simulink model "sysgenPBDemo"  (Simulink 7.7)
settings: Solver=ode45  StartTime=0.0  StopTime=500  RelTol=1e-3
libraries: xbsIndex_r4 x19, xbsCopyrightNotice_r4 x1
settings Model: Creator=alexc  LastModifiedBy=arvinds
settings DataIOCC: SignalLoggingName=sigsOut
settings OptimizationCC: BooleanDataType=off  InlineInvariantSignals=on  InitFltsAndDblsToZero=on
settings DebuggingCC: SaveWithParameterizedLinksMsg=none  SignalResolutionControl=TryResolveAllWithWarning  SolverPrmCheckMsg=none  MultiTaskDSMMsg=warning  MultiTaskCondExecSysMsg=none  StrictBusMsg=None
settings HardwareCC: TargetUnknown=on
settings RTWCC: IncludeERTFirstTime=on
settings GRTTargetCC: TargetFcnLib=ansi_tfl_tmw.mat

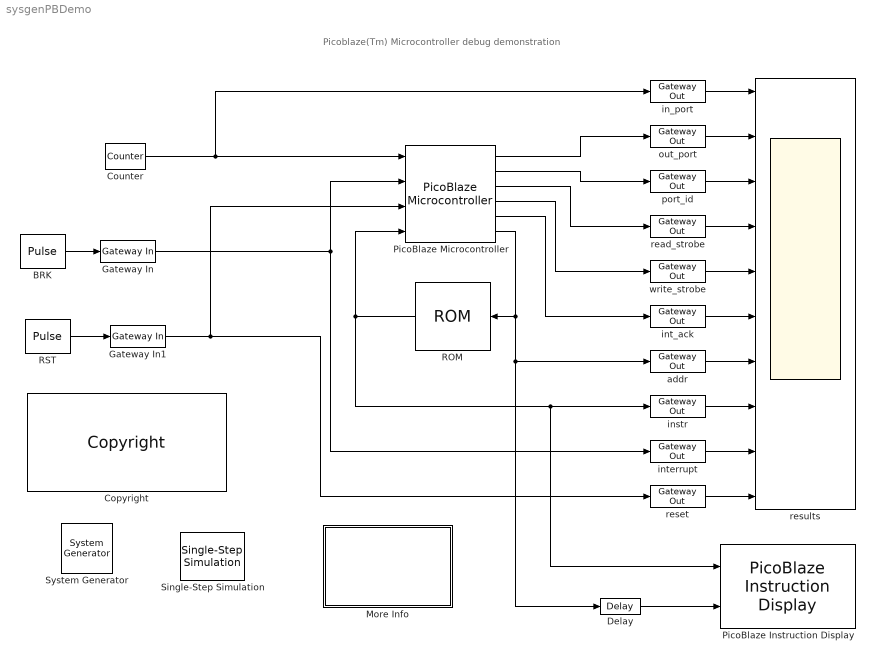
== system sysgenPBDemo ==
  note: Picoblaze(Tm) Microcontroller debug demonstration
  " System Generator" : xbsIndex_r4/ System Generator  Tag=genX  SystemSampleTime=-1  xilinxfamily=virtex4  part=xc4vlx200  speed=-11  package=ff1513  synthesis_tool=XST  clock_wrapper=Clock Enables  directory=C:/sb/demos/byhandtest/sysgenPBDemo  proj_type=Project Navigator  Synth_file=XST Defaults  Impl_file=ISE Defaults  testbench=on  simulink_period=1  sysclk_period=100  dcm_input_clock_period=100  incr_netlist=off  trim_vbits=Everywhere in SubSystem  dbl_ovrd=According to Block Masks  core_generation=According to Block Masks  run_coregen=off  deprecated_control=off  eval_field=0  block_type=sysgen
      settings: block_version=10.1.00
  BRK : DiscretePulseGenerator  Period=1000  PulseWidth=2
  Copyright : xbsCopyrightNotice_r4/Copyright  copyrighttext="Copyright (c) 2011  by  Xilinx, Inc. All rights reserved.<br><br>This file contains proprietary, confidential information of Xilinx, Inc., is distributed under license from Xilinx, Inc., and may be used, copied and/or disclosed only pursuant to the terms of a valid license agreement with Xilinx, Inc. Xilinx hereby grants you a license to use this file solely for design, simulation, implementation and creation of design files limited to Xilinx devices or technologies. Use with non-Xilinx devices or technologies is expressly prohibited and immediately terminates your license unless covered by a separate agreement.<br><br>Xilinx is providing this design, code, or information \"as-is\" solely for use in developing programs and solutions for Xilinx devices, with no obligation on the part of Xilinx to provide support. By providing this design, code, or information as one possible implementation of this feature, application or standard, Xilinx is making no representation that this implementation is free from any claims of infringement. You are responsible for obtaining any rights you may require for your implementation. Xilinx expressly disclaims any warranty whatsoever with respect to the adequacy of the implementation, including but not limited to any warranties or representations that this implementation is free from claims of infringement, implied warranties of merchantability or fitness for a particular purpose.<br><br>Xilinx products are not intended for use in life support appliances, devices, or systems. Use in such applications is expressly prohibited.<br><br>Any modifications that are made to the Source Code are done at the user's sole risk and will be unsupported.<br><br>This copyright and support notice must be retained as part of this text at all times. (c) Copyright 1995-2011 Xilinx, Inc. All rights reserved."  block_type=copyright
      settings: block_version=10.1.00
      settings: infoedit=|
      | Copyright(C) 2008 by  Xilinx, Inc. All rights reserved.<br>
      | <br>
      | This file contains proprietary, confidential information of Xilinx, Inc., is distributed under license
      | from Xilinx, Inc., and may be used, copied and/or disclosed only pursuant to the terms of a valid license
      | agreement with Xilinx, Inc. Xilinx hereby grants you a license to use this file solely for design,
      | simulation, implementation and creation of design files limited to Xilinx devices or technologies. Use
      | with non-Xilinx devices or technologies is expressly prohibited and immediately terminates your license
      | unless covered by a separate agreement.<br>
      | <br>
      | Xilinx is providing this design, code, or information "as-is" solely for use in developing programs and
      | solutions for Xilinx devices, with no obligation on the part of Xilinx to provide support. By providing
      | this design, code, or information as one possible implementation of this feature, application or standard,
      | Xilinx is making no representation that this implementation is free from any claims of infringement. You
      | are responsible for obtaining any rights you may require for your implementation. Xilinx expressly disclaims
      | any warranty whatsoever with respect to the adequacy of the implementation, including but not limited to any
      | warranties or representations that this implementation is free from claims of infringement, implied warranties
      | of merchantability or fitness for a particular purpose.<br>
      | <br>
      | Xilinx products are not intended for use in life support appliances, devices, or systems. Use in such
      | applications is expressly prohibited.<br>
      | <br>
      | Any modifications that are made to the Source Code are done at the user's sole risk and will be unsupported.<br>
      | <br>
      | This copyright and support notice must be retained as part of this text at all times.
      | (c) Copyright 1995-2008 Xilinx, Inc. All rights reserved.
  Counter : xbsIndex_r4/Counter  cnt_type=Count Limited  cnt_to=Inf  operation=Up  start_count=0  cnt_by_val=1  arith_type=Unsigned  n_bits=8  bin_pt=0  load_pin=off  rst=off  en=off  explicit_period=off  period=1  dbl_ovrd=off  use_behavioral_HDL=off  implementation=Fabric  use_rpm=off  block_type=counter
      settings: xl_area=[0, 0, 0, 0, 0, 0, 0]  block_version=VER_STRING_GOES_HERE
  Delay : xbsIndex_r4/Delay  rst=off  infoeditControl=Selection of Reset will increase slice count due to use of real FFs and instead of SRLs  en=off  latency=1  dbl_ovrd=off  reg_retiming=off  block_type=delay
      settings: infoedit=Hardware notes: A delay line is a chain, each link of which is an SRL16 followed by a flip-flop. If register retiming is enabled, the delay line is a chain of flip-flops.  xl_area=[0, 0, 0, 0, 0, 0, 0]  block_version=VER_STRING_GOES_HERE
  Gateway In : xbsIndex_r4/Gateway In  gui_display_data_type=Fixed-point  arith_type=Boolean  n_bits=8  bin_pt=6  preci_type=Single  exp_width=8  frac_width=24  quantization="Round  (unbiased: +/- Inf)"  overflow=Saturate  period=1  dbl_ovrd=off  timing_constraint=None  locs_specified=off  LOCs={}  hdl_port=on  block_type=gatewayin
      settings: infoedit="Gateway in block.  Converts inputs of type Simulink integer, double and fixed point to  Xilinx fixed point type.<P><P>Hardware notes:  In hardware these blocks become top level input ports."  xl_area=[0, 0, 0, 0, 0, 0, 0]  block_version=VER_STRING_GOES_HERE
  Gateway In1 : xbsIndex_r4/Gateway In  gui_display_data_type=Fixed-point  arith_type=Boolean  n_bits=8  bin_pt=6  preci_type=Single  exp_width=8  frac_width=24  quantization="Round  (unbiased: +/- Inf)"  overflow=Saturate  period=1  dbl_ovrd=off  timing_constraint=None  locs_specified=off  LOCs={}  hdl_port=on  block_type=gatewayin
      settings: infoedit="Gateway in block.  Converts inputs of type Simulink integer, double and fixed point to  Xilinx fixed point type.<P><P>Hardware notes:  In hardware these blocks become top level input ports."  xl_area=[0, 0, 0, 0, 0, 0, 0]  block_version=VER_STRING_GOES_HERE
  More Info : Subsystem
      mask Display: disp('Double click\n for\n more information.')
  PicoBlaze Microcontroller : xbsIndex_r4/PicoBlaze Microcontroller  version=PicoBlaze 3  display_mi=on  xl_view_as=Decimal  block_type=pb
      settings: xl_area=[0, 0, 0, 0, 0, 0, 0]  block_version=VER_STRING_GOES_HERE
  PicoBlaze Instruction Display : xbsIndex_r4/PicoBlaze Instruction Display  SystemSampleTime=-1  xl_pb_inst=OUTPUT sE, 14  xl_pb_pc=54  xl_pb_version=PicoBlaze 3  xl_pb_disable=off  block_type=picoblazeinstr
      settings: infoedit=PicoBlaze Instruction\nDisplay  block_version=10.1.00
  ROM : xbsIndex_r4/ROM  depth=1024  initVector=fill_pbdemo_program_store  distributed_mem=Block RAM  rst=off  init_reg=0  en=off  latency=1  gui_display_data_type=Fixed-point  arith_type=Unsigned  n_bits=18  bin_pt=0  preci_type=Single  exp_width=8  frac_width=24  dbl_ovrd=off  optimize=Area  use_rpm=off  block_type=sprom
      settings: xl_area=[0, 0, 0, 0, 0, 0, 0]  block_version=VER_STRING_GOES_HERE
  RST : DiscretePulseGenerator  Period=3000  PulseWidth=2
  Single-Step Simulation : xbsIndex_r4/Single-Step Simulation  SystemSampleTime=-1  xl_status=Continuous  xl_state=1  block_type=singlestep
      settings: infoedit=Single-Step\nSimulation  block_version=10.1.00
  addr : xbsIndex_r4/Gateway Out  hdl_port=on  timing_constraint=None  locs_specified=off  LOCs={}  block_type=gatewayout
      settings: infoedit="Gateway out block.  Converts Xilinx fixed point inputs into ouputs of type Simulink integer, double, or fixed point.<P><P>Hardware notes:  In hardware these blocks become top level output ports or are discarded, depending on how they are configured."  xl_area=[0, 0, 0, 0, 0, 0, 0]  block_version=VER_STRING_GOES_HERE
  in_port : xbsIndex_r4/Gateway Out  hdl_port=on  timing_constraint=None  locs_specified=off  LOCs={}  block_type=gatewayout
      settings: infoedit="Gateway out block.  Converts Xilinx fixed point inputs into ouputs of type Simulink integer, double, or fixed point.<P><P>Hardware notes:  In hardware these blocks become top level output ports or are discarded, depending on how they are configured."  xl_area=[0, 0, 0, 0, 0, 0, 0]  block_version=VER_STRING_GOES_HERE
  instr : xbsIndex_r4/Gateway Out  hdl_port=on  timing_constraint=None  locs_specified=off  LOCs={}  block_type=gatewayout
      settings: infoedit="Gateway out block.  Converts Xilinx fixed point inputs into ouputs of type Simulink integer, double, or fixed point.<P><P>Hardware notes:  In hardware these blocks become top level output ports or are discarded, depending on how they are configured."  xl_area=[0, 0, 0, 0, 0, 0, 0]  block_version=VER_STRING_GOES_HERE
  int_ack : xbsIndex_r4/Gateway Out  hdl_port=on  timing_constraint=None  locs_specified=off  LOCs={}  block_type=gatewayout
      settings: infoedit="Gateway out block.  Converts Xilinx fixed point inputs into ouputs of type Simulink integer, double, or fixed point.<P><P>Hardware notes:  In hardware these blocks become top level output ports or are discarded, depending on how they are configured."  xl_area=[0, 0, 0, 0, 0, 0, 0]  block_version=VER_STRING_GOES_HERE
  interrupt : xbsIndex_r4/Gateway Out  hdl_port=on  timing_constraint=None  locs_specified=off  LOCs={}  block_type=gatewayout
      settings: infoedit="Gateway out block.  Converts Xilinx fixed point inputs into ouputs of type Simulink integer, double, or fixed point.<P><P>Hardware notes:  In hardware these blocks become top level output ports or are discarded, depending on how they are configured."  xl_area=[0, 0, 0, 0, 0, 0, 0]  block_version=VER_STRING_GOES_HERE
  out_port : xbsIndex_r4/Gateway Out  hdl_port=on  timing_constraint=None  locs_specified=off  LOCs={}  block_type=gatewayout
      settings: infoedit="Gateway out block.  Converts Xilinx fixed point inputs into ouputs of type Simulink integer, double, or fixed point.<P><P>Hardware notes:  In hardware these blocks become top level output ports or are discarded, depending on how they are configured."  xl_area=[0, 0, 0, 0, 0, 0, 0]  block_version=VER_STRING_GOES_HERE
  port_id : xbsIndex_r4/Gateway Out  hdl_port=on  timing_constraint=None  locs_specified=off  LOCs={}  block_type=gatewayout
      settings: infoedit="Gateway out block.  Converts Xilinx fixed point inputs into ouputs of type Simulink integer, double, or fixed point.<P><P>Hardware notes:  In hardware these blocks become top level output ports or are discarded, depending on how they are configured."  xl_area=[0, 0, 0, 0, 0, 0, 0]  block_version=VER_STRING_GOES_HERE
  read_strobe : xbsIndex_r4/Gateway Out  hdl_port=on  timing_constraint=None  locs_specified=off  LOCs={}  block_type=gatewayout
      settings: infoedit="Gateway out block.  Converts Xilinx fixed point inputs into ouputs of type Simulink integer, double, or fixed point.<P><P>Hardware notes:  In hardware these blocks become top level output ports or are discarded, depending on how they are configured."  xl_area=[0, 0, 0, 0, 0, 0, 0]  block_version=VER_STRING_GOES_HERE
  reset : xbsIndex_r4/Gateway Out  hdl_port=on  timing_constraint=None  locs_specified=off  LOCs={}  block_type=gatewayout
      settings: infoedit="Gateway out block.  Converts Xilinx fixed point inputs into ouputs of type Simulink integer, double, or fixed point.<P><P>Hardware notes:  In hardware these blocks become top level output ports or are discarded, depending on how they are configured."  xl_area=[0, 0, 0, 0, 0, 0, 0]  block_version=VER_STRING_GOES_HERE
  results : Scope  NumInputPorts=10
      settings: TickLabels=on  YMin=6~6~-5~-0.1~-0.1~0~0~-0.1~-0.1~-0.1  YMax=9~9~5~1.5~1.5~30~300000~1.5~1.2~1.5
  write_strobe : xbsIndex_r4/Gateway Out  hdl_port=on  timing_constraint=None  locs_specified=off  LOCs={}  block_type=gatewayout
      settings: infoedit="Gateway out block.  Converts Xilinx fixed point inputs into ouputs of type Simulink integer, double, or fixed point.<P><P>Hardware notes:  In hardware these blocks become top level output ports or are discarded, depending on how they are configured."  xl_area=[0, 0, 0, 0, 0, 0, 0]  block_version=VER_STRING_GOES_HERE
  wires:
  PicoBlaze Microcontroller/1 -> out_port/1
  PicoBlaze Microcontroller/2 -> port_id/1
  PicoBlaze Microcontroller/3 -> read_strobe/1
  PicoBlaze Microcontroller/4 -> write_strobe/1
  out_port/1 -> results/2
  port_id/1 -> results/3
  read_strobe/1 -> results/4
  write_strobe/1 -> results/5
  in_port/1 -> results/1
  Counter/1 -> in_port/1, PicoBlaze Microcontroller/1
  Gateway In/1 -> interrupt/1, PicoBlaze Microcontroller/2
  Gateway In1/1 -> PicoBlaze Microcontroller/3, reset/1
  RST/1 -> Gateway In1/1
  BRK/1 -> Gateway In/1
  Delay/1 -> PicoBlaze Instruction Display/2
  ROM/1 -> PicoBlaze Microcontroller/4, instr/1, PicoBlaze Instruction Display/1
  PicoBlaze Microcontroller/6 -> ROM/1, Delay/1, addr/1
  int_ack/1 -> results/6
  PicoBlaze Microcontroller/5 -> int_ack/1
  addr/1 -> results/7
  instr/1 -> results/8
  interrupt/1 -> results/9
  reset/1 -> results/10

== system sysgenPBDemo/More Info ==
  note: Picoblaze(Tm) Microcontroller debug demonstration
  note: This model shows how to debug a design containing
      | the PicoBlaze(tm) microcontroller.  The debugging tools
      | allow simulations to single-step or run continuously,
      | display microcontroller internals, and show which
      | instruction is being executed at the moment.
      |
      | To make the simulation run continuously, flip the switch
      | driving "Single-Step Simulation"  up; when the switch
      | is up, the simulation pauses after every clock cycle.
      | Note each microcontroller instruction takes two cycles.
      | The block named "PicoBlaze Instruction Display" shows
      | which instruction is executing at the moment.  The
      | microcontroller itself is inside the subsystem named
      | "Microcontroller Subsystem".  Turning on the
      | microcontroller's  "Display Microcontroller Internals"
      | checkbox causes internal values to be made visible.
      |
      | The single step simulation and instruction display blocks
      | can be used in any model that includes a PicoBlaze(tm)
      | microcontroller - simply copy the blocks into the model.
